simulink model "modFerObser"  (R2016b)
settings: Solver=VariableStepAuto  StartTime=0.0  StopTime=100  RelTol=1e-3  EnableMultiTasking=on
values from neighbouring files (symbols this model uses):
  A = [ 0   0  0 ... (first row only)    [detectability.m]    (also in param.m = [-0.02   1    1)
  Aob = A-L*C    [param.m]
  B = [1.6;0.23;0]    [param.m]
  Bob = [B L]    [param.m]
  C = [ 0 0 0]    [detectability.m]    (also in param.m = [1 0 0])
  Cob = eye(3)    [param.m]
  Dob = zeros(3,2)    [param.m]
  K1lqr = Klqr(1:3)    [param.m]
  Kslqr = Klqr(4)    [param.m]
settings Model: Creator=ganou2u  LastModifiedBy=arek
settings OptimizationCC: LifeSpan=inf
settings DebuggingCC: SFUnexpectedBacktrackingDiag=warning  SFNoUnconditionalDefaultTransitionDiag=warning  SFExecutionAtInitializationDiag=none
settings GRTTargetCC: TargetLangStandard=C89/C90 (ANSI)  GeneratePreprocessorConditionals=Disable all
settings ConfigComp: CovMetricSettings=dw  CovHtmlReporting=on  CovSaveCumulativeToWorkspaceVar=on  CovSaveSingleToWorkspaceVar=on  CovExternalEMLEnable=off

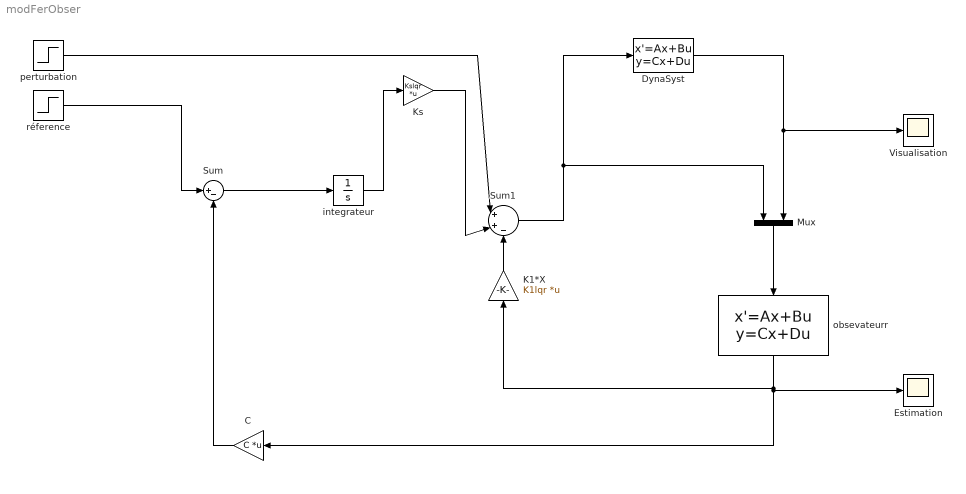
== system modFerObser ==
  C : Gain  Gain=C  Multiplication=Matrix(K*u)
  DynaSyst : StateSpace  A=A  B=B  C=C  D=0  X0=0
  Estimation : Scope
  K1*X : Gain  Gain=K1lqr  Multiplication=Matrix(K*u)
  Ks : Gain  Gain=Kslqr  Multiplication=Matrix(K*u)
  Mux : Mux  Inputs=2
  Sum : Sum  Inputs=|+-
  Sum1 : Sum  Inputs=|++-
  Visualisation : Scope
  integrateur : Integrator
  obsevateurr : StateSpace  A=Aob  B=Bob  C=Cob  D=Dob  X0=0
  perturbation : Step  Time=5  After=20  SampleTime=0
  réference : Step  Time=0  SampleTime=0
  wires:
  réference/1 -> Sum/1
  DynaSyst/1 -> Mux/2, Visualisation/1
  Sum1/1 -> Mux/1, DynaSyst/1
  Sum/1 -> integrateur/1
  integrateur/1 -> Ks/1
  Ks/1 -> Sum1/2
  K1*X/1 -> Sum1/3
  obsevateurr/1 -> Estimation/1, C/1, K1*X/1
  Mux/1 -> obsevateurr/1
  C/1 -> Sum/2
  perturbation/1 -> Sum1/1
